simulink model "RightCameraAgent"  (Simulink 6.2)
settings: Solver=ode45  StartTime=0.0  StopTime=10.0  RelTol=1e-3
settings Model: LastModifiedBy=suarezjl
settings DataIOCC: SignalLoggingName=sigsOut
settings HardwareCC: TargetUnknown=on

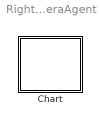
== system RightCameraAgent ==
  Chart : Stateflow chart

== stateflow chart Chart ==
  state Initial
    \\Sally\HeadTrackingDemo\RightCameraAgent\FrameGrabber.Initialize()
    \\Sally\HeadTrackingDemo\RightCameraAgent\FrameGrabber.ObtainImage()
    \\Sally\HeadTrackingDemo\RightCameraAgent\FrameGrabber.ObtainImage()
    \\Sally\HeadTrackingDemo\RightCameraAgent\ColorSegmenter.Initial()
    \\Sally\HeadTrackingDemo\RightCameraAgent\ColorSegmenter.LoadColorModel()
  state Segmentation
    \\Sally\HeadTrackingDemo\RightCameraAgent\FrameGrabber.ObtainImage()
    \\Sally\HeadTrackingDemo\RightCameraAgent\ColorSegmenter.DoSegment()
  (default) -> Initial : Start
  Initial -> Segmentation : Always
  Segmentation -> Segmentation : Always
